simulink model "ME3360_Project1_e"  (R2018b)
settings: Solver=VariableStepAuto  StartTime=0.0  StopTime=200  RelTol=1e-3
values from neighbouring files (symbols this model uses):
  b = 62    [Part1_d.m]    (also in Part1_e.m)
  d = 0.48    [Part1_d.m]    (also in Part1_e.m)
  g = 9.81    [Part1_e.m]
  m = 2110    [Part1_d.m]    (also in Part1_e.m)
  theta = 3    [Part1_e.m]
  Tmax = 1465    [Part1_d.m]    (also in Part1_e.m)
  Tss = 99.8    [Part1_d.m]    (also in Part1_e.m)
settings Model: Creator=Andrew  LastModifiedBy=Nick Carcione

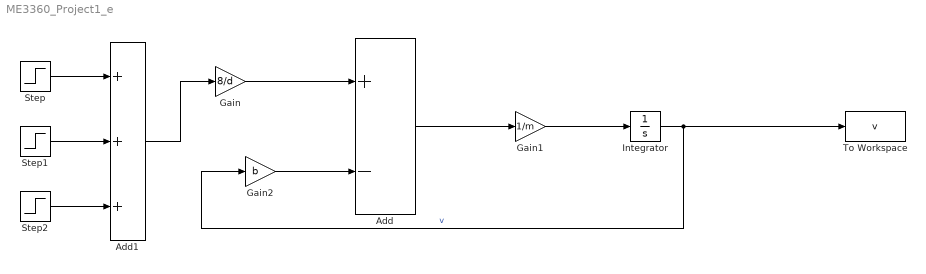
== system ME3360_Project1_e ==
  Add : Sum  Inputs=+-
  Add1 : Sum  Inputs=+++
  Gain : Gain  Gain=8/d
  Gain1 : Gain  Gain=1/m
  Gain2 : Gain  Gain=b
  Integrator : Integrator
  Step : Step  Time=0  After=Tmax  SampleTime=0
  Step1 : Step  Time=2.4  After=Tss-Tmax  SampleTime=0
  Step2 : Step  Time=10  After=m*g*cosd(theta)*Tss-Tss  SampleTime=0
  To Workspace : ToWorkspace  VariableName=v  SaveFormat=Timeseries  SampleTime=-1
  wires:
  Integrator/1 -> To Workspace/1, Gain2/1  "v"
  Gain1/1 -> Integrator/1
  Add/1 -> Gain1/1
  Step2/1 -> Add1/3
  Step1/1 -> Add1/2
  Step/1 -> Add1/1
  Add1/1 -> Gain/1
  Gain2/1 -> Add/2
  Gain/1 -> Add/1
